simulink model "PSK"  (R2023b)
settings: Solver=VariableStepAuto  StartTime=0.0  StopTime=10.0  RelTol=1e-3
settings Model: Creator=satyamagrawal  LastModifiedBy=satyamagrawal

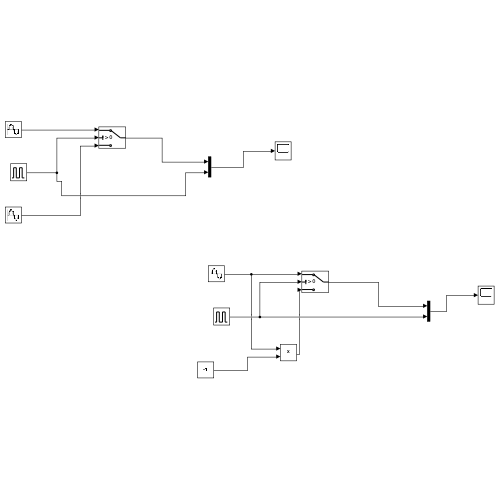
[thumbnail: Simulink's stored preview of the top-level diagram]
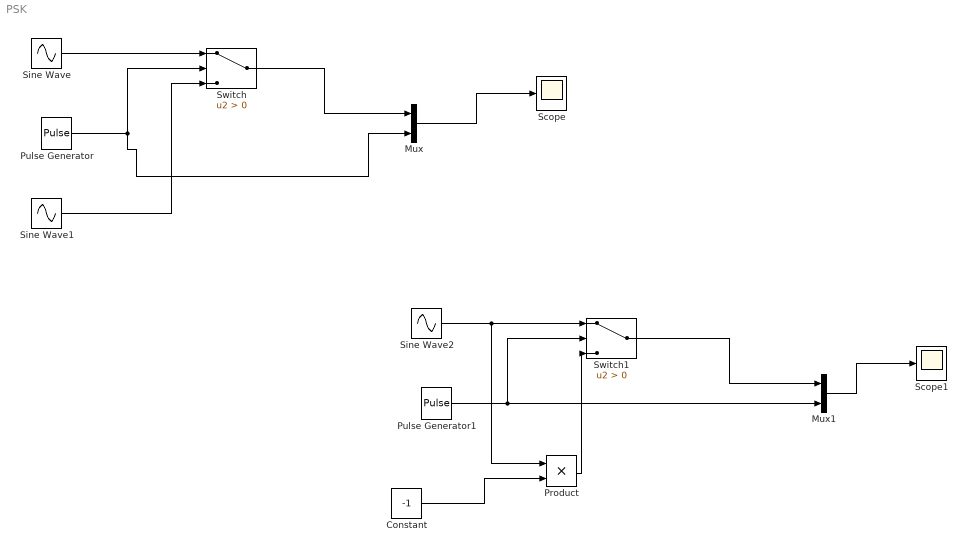
== system PSK ==
  Constant : Constant  Value=-1
  Mux : Mux  Inputs=2
  Mux1 : Mux  Inputs=2
  Product : Product
  Pulse Generator : DiscretePulseGenerator  PulseType=Time based  Period=10  PulseWidth=50
  Pulse Generator1 : DiscretePulseGenerator  PulseType=Time based  Period=5  PulseWidth=50
  Scope : Scope
  Scope1 : Scope
  Sine Wave : Sin  Frequency=6  SampleTime=0.00001
  Sine Wave1 : Sin  Frequency=6  Phase=pi  SampleTime=0.00001
  Sine Wave2 : Sin  Frequency=10  SampleTime=0.001
  Switch : Switch  Criteria=u2 > Threshold  SaturateOnIntegerOverflow=off  InputSameDT=off
  Switch1 : Switch  Criteria=u2 > Threshold  SaturateOnIntegerOverflow=off  InputSameDT=off
  wires:
  Switch/1 -> Mux/1
  Pulse Generator/1 -> Mux/2, Switch/2
  Sine Wave1/1 -> Switch/3
  Sine Wave/1 -> Switch/1
  Mux/1 -> Scope/1
  Switch1/1 -> Mux1/1
  Pulse Generator1/1 -> Switch1/2, Mux1/2
  Sine Wave2/1 -> Product/1, Switch1/1
  Mux1/1 -> Scope1/1
  Constant/1 -> Product/2
  Product/1 -> Switch1/3
